simulink model "TD"  (R2018a)
settings: Solver=VariableStepAuto  StartTime=0.0  StopTime=20.0  RelTol=1e-3
libraries: simulink x5
settings Model: Creator=Administrator  LastModifiedBy=Administrator
settings SolverCC: ZeroCrossAlgorithm=Adaptive
settings DebuggingCC: MaxConsecutiveZCsMsg=none  IgnoredZcDiagnostic=none

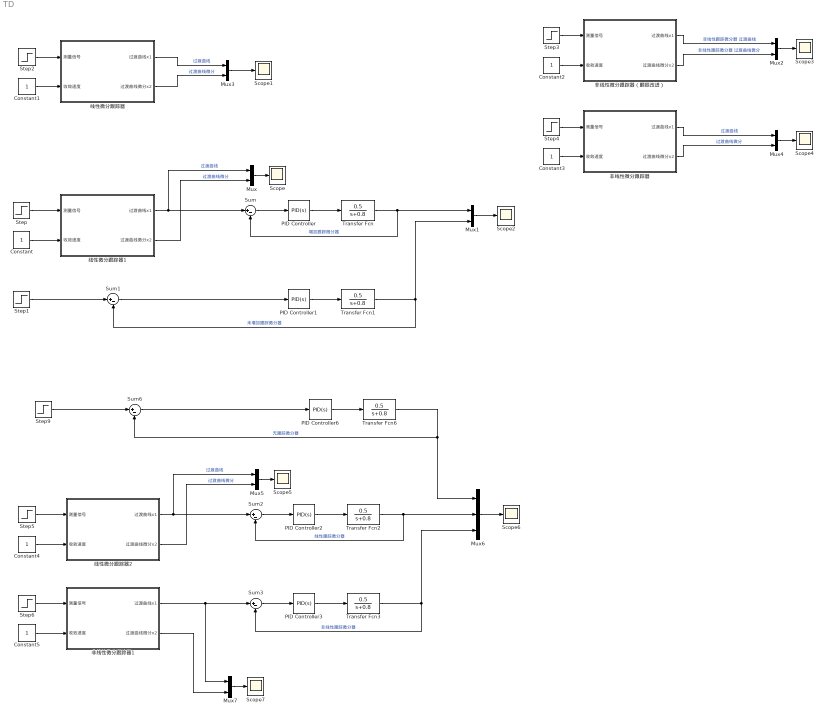
== system TD ==
  Constant{,1..5} (6 alike) : Constant
  Mux{,1..5,7} (7 alike) : Mux  Inputs=2
  Mux6 : Mux  Inputs=3
  PID Controller{,1..3,6} (5 alike) : simulink/Continuous/PID Controller  Controller=PID  TimeDomain=Continuous-time  SampleTime=-1  IntegratorMethod=Forward Euler  FilterMethod=Forward Euler  Form=Parallel  UseFilter=on  ControllerParametersSource=internal  P=10  I=10  D=1  N=100  InitialConditionSource=internal  InitialConditionForIntegrator=0  InitialConditionForFilter=0  ExternalReset=none  LimitOutput=off  UpperSaturationLimit=inf  LowerSaturationLimit=-inf  LinearizeAsGain=on  AntiWindupMode=none  Kb=1  TrackingMode=off  Kt=1  PParamMin=[]  PParamMax=[]  IParamMin=[]  IParamMax=[]  DParamMin=[]  DParamMax=[]  NParamMin=[]  NParamMax=[]  KbParamMin=[]  KbParamMax=[]  KtParamMin=[]  KtParamMax=[]  POutMin=[]  POutMax=[]  IOutMin=[]  IOutMax=[]  DOutMin=[]  DOutMax=[]  NOutMin=[]  NOutMax=[]  KbOutMin=[]  KbOutMax=[]  KtOutMin=[]  KtOutMax=[]  IntegratorOutMin=[]  IntegratorOutMax=[]  FilterOutMin=[]  FilterOutMax=[]  SumOutMin=[]  SumOutMax=[]  SumI1OutMin=[]  SumI1OutMax=[]  SumI2OutMin=[]  SumI2OutMax=[]  SumI3OutMin=[]  SumI3OutMax=[]  SumDOutMin=[]  SumDOutMax=[]  SaturationOutMin=[]  SaturationOutMax=[]  IntegratorContinuousStateAttributes=''  IntegratorStateMustResolveToSignalObject=off  IntegratorRTWStateStorageClass=Auto  FilterContinuousStateAttributes=''  FilterStateMustResolveToSignalObject=off  FilterRTWStateStorageClass=Auto  DifferentiatorICPrevScaledInput=0  DifferentiatorOutMin=[]  DifferentiatorOutMax=[]  FilterDiffOutCoefMin=[]  FilterDiffOutCoefMax=[]  SumDenOutMin=[]  SumDenOutMax=[]  SumNumOutMin=[]  SumNumOutMax=[]  ReciprocalOutMin=[]  ReciprocalOutMax=[]  DivideOutMin=[]  DivideOutMax=[]  TunerSelectOption=Transfer Function Based (PID Tuner App)
  Scope{,1..7} (8 alike) : Scope
  Step{,1..6,9} (8 alike) : Step  SampleTime=0
  Sum{,1..3,6} (5 alike) : Sum  Inputs=|+-
  Transfer Fcn{,1..3,6} (5 alike) : TransferFcn  Numerator=[0.5]  Denominator=[1 0.8]
  线性微分跟踪器 : Subsystem
  线性微分跟踪器1 : Subsystem
  线性微分跟踪器2 : Subsystem
  非线性微分跟踪器 : Subsystem
  非线性微分跟踪器1 : Subsystem
  非线性微分跟踪器（颤振改进） : Subsystem
  wires:
  Step/1 -> 线性微分跟踪器1/1(测量信号)
  Constant/1 -> 线性微分跟踪器1/2(收敛速度)
  线性微分跟踪器1/1(过渡曲线x1) -> Sum/1, Mux/1  "过渡曲线"
  线性微分跟踪器1/2(过渡曲线微分x2) -> Mux/2  "过渡曲线微分"
  Sum/1 -> PID Controller/1
  Mux/1 -> Scope/1
  PID Controller/1 -> Transfer Fcn/1
  PID Controller1/1 -> Transfer Fcn1/1
  Sum1/1 -> PID Controller1/1
  Transfer Fcn/1 -> Sum/2, Mux1/1  "增加跟踪微分器"
  Step2/1 -> 线性微分跟踪器/1(测量信号)
  Constant1/1 -> 线性微分跟踪器/2(收敛速度)
  线性微分跟踪器/1(过渡曲线x1) -> Mux3/1  "过渡曲线"
  线性微分跟踪器/2(过渡曲线微分x2) -> Mux3/2  "过渡曲线微分"
  Mux3/1 -> Scope1/1
  Transfer Fcn1/1 -> Sum1/2, Mux1/2  "未增加跟踪微分器"
  Step1/1 -> Sum1/1
  Mux1/1 -> Scope2/1
  Constant2/1 -> 非线性微分跟踪器（颤振改进）/2(收敛速度)
  Step3/1 -> 非线性微分跟踪器（颤振改进）/1(测量信号)
  Mux2/1 -> Scope3/1
  非线性微分跟踪器（颤振改进）/2(过渡曲线微分x2) -> Mux2/2  "非线性跟踪微分器 过渡曲线微分"
  非线性微分跟踪器（颤振改进）/1(过渡曲线x1) -> Mux2/1  "非线性跟踪微分器 过渡曲线"
  非线性微分跟踪器/1(过渡曲线x1) -> Mux4/1  "过渡曲线"
  非线性微分跟踪器/2(过渡曲线微分x2) -> Mux4/2  "过渡曲线微分"
  Constant3/1 -> 非线性微分跟踪器/2(收敛速度)
  Mux4/1 -> Scope4/1
  Step4/1 -> 非线性微分跟踪器/1(测量信号)
  Constant4/1 -> 线性微分跟踪器2/2(收敛速度)
  Step5/1 -> 线性微分跟踪器2/1(测量信号)
  线性微分跟踪器2/1(过渡曲线x1) -> Sum2/1, Mux5/1  "过渡曲线"
  线性微分跟踪器2/2(过渡曲线微分x2) -> Mux5/2  "过渡曲线微分"
  Mux6/1 -> Scope6/1
  PID Controller2/1 -> Transfer Fcn2/1
  Transfer Fcn3/1 -> Sum3/2, Mux6/3  "非线性跟踪微分器"
  Sum2/1 -> PID Controller2/1
  Sum3/1 -> PID Controller3/1
  PID Controller3/1 -> Transfer Fcn3/1
  Transfer Fcn2/1 -> Sum2/2, Mux6/2  "线性跟踪微分器"
  非线性微分跟踪器1/1(过渡曲线x1) -> Mux7/1, Sum3/1
  Mux5/1 -> Scope5/1
  Step6/1 -> 非线性微分跟踪器1/1(测量信号)
  Constant5/1 -> 非线性微分跟踪器1/2(收敛速度)
  非线性微分跟踪器1/2(过渡曲线微分x2) -> Mux7/2
  Mux7/1 -> Scope7/1
  Sum6/1 -> PID Controller6/1
  PID Controller6/1 -> Transfer Fcn6/1
  Transfer Fcn6/1 -> Mux6/1, Sum6/2  "无跟踪微分器"
  Step9/1 -> Sum6/1

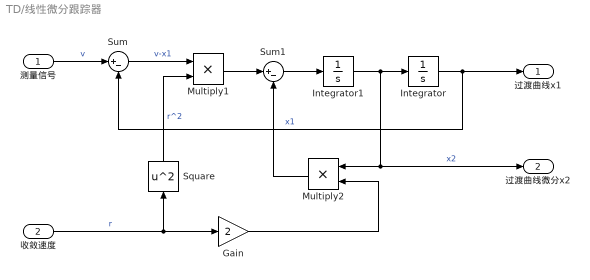
== system TD/线性微分跟踪器 ==
  测量信号 : Inport
  收敛速度 : Inport  Port=2
  Gain : Gain  Gain=2
  Integrator : Integrator
  Integrator1 : Integrator
  Multiply1 : Product
  Multiply2 : Product
  Square : Math  Operator=square  SaturateOnIntegerOverflow=on
  Sum : Sum  Inputs=|+-
  Sum1 : Sum  Inputs=|+-
  过渡曲线x1 : Outport
  过渡曲线微分x2 : Outport  Port=2
  wires:
  Integrator/1 -> 过渡曲线x1/1, Sum/2  "x1"
  Multiply2/1 -> Sum1/2
  Integrator1/1 -> Integrator/1, Multiply2/1, 过渡曲线微分x2/1  "x2"
  测量信号/1 -> Sum/1  "v"
  Multiply1/1 -> Sum1/1
  Sum1/1 -> Integrator1/1
  Gain/1 -> Multiply2/2
  Sum/1 -> Multiply1/1  "v-x1"
  收敛速度/1 -> Square/1, Gain/1  "r"
  Square/1 -> Multiply1/2  "r^2"

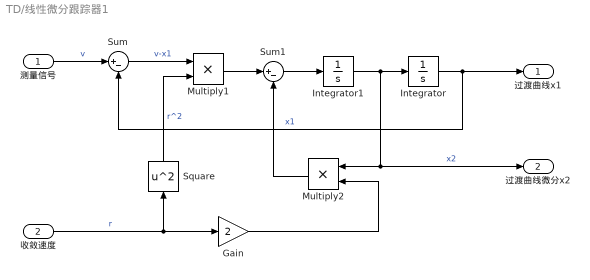
== system TD/线性微分跟踪器1 ==
  测量信号 : Inport
  收敛速度 : Inport  Port=2
  Gain : Gain  Gain=2
  Integrator : Integrator
  Integrator1 : Integrator
  Multiply1 : Product
  Multiply2 : Product
  Square : Math  Operator=square  SaturateOnIntegerOverflow=on
  Sum : Sum  Inputs=|+-
  Sum1 : Sum  Inputs=|+-
  过渡曲线x1 : Outport
  过渡曲线微分x2 : Outport  Port=2
  wires:
  Integrator/1 -> 过渡曲线x1/1, Sum/2  "x1"
  Multiply2/1 -> Sum1/2
  Integrator1/1 -> Integrator/1, Multiply2/1, 过渡曲线微分x2/1  "x2"
  测量信号/1 -> Sum/1  "v"
  Multiply1/1 -> Sum1/1
  Sum1/1 -> Integrator1/1
  Gain/1 -> Multiply2/2
  Sum/1 -> Multiply1/1  "v-x1"
  收敛速度/1 -> Square/1, Gain/1  "r"
  Square/1 -> Multiply1/2  "r^2"

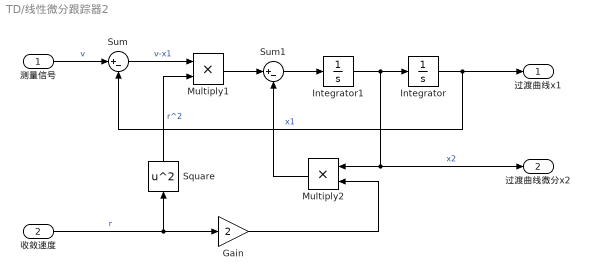
== system TD/线性微分跟踪器2 ==
  测量信号 : Inport
  收敛速度 : Inport  Port=2
  Gain : Gain  Gain=2
  Integrator : Integrator
  Integrator1 : Integrator
  Multiply1 : Product
  Multiply2 : Product
  Square : Math  Operator=square  SaturateOnIntegerOverflow=on
  Sum : Sum  Inputs=|+-
  Sum1 : Sum  Inputs=|+-
  过渡曲线x1 : Outport
  过渡曲线微分x2 : Outport  Port=2
  wires:
  Integrator/1 -> 过渡曲线x1/1, Sum/2  "x1"
  Multiply2/1 -> Sum1/2
  Integrator1/1 -> Integrator/1, Multiply2/1, 过渡曲线微分x2/1  "x2"
  测量信号/1 -> Sum/1  "v"
  Multiply1/1 -> Sum1/1
  Sum1/1 -> Integrator1/1
  Gain/1 -> Multiply2/2
  Sum/1 -> Multiply1/1  "v-x1"
  收敛速度/1 -> Square/1, Gain/1  "r"
  Square/1 -> Multiply1/2  "r^2"

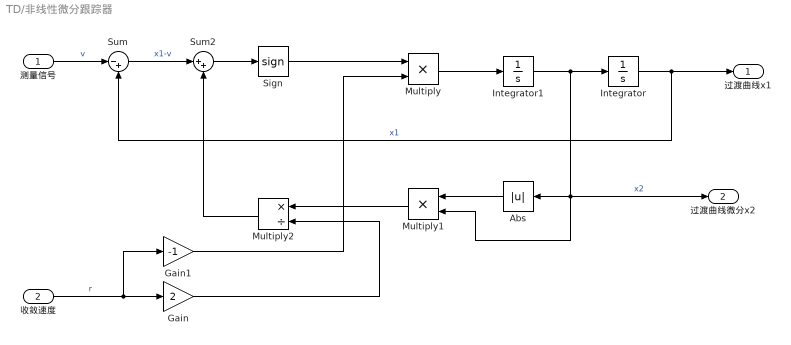
== system TD/非线性微分跟踪器 ==
  测量信号 : Inport
  收敛速度 : Inport  Port=2
  Abs : Abs
  Gain : Gain  Gain=2
  Gain1 : Gain  Gain=-1
  Integrator : Integrator
  Integrator1 : Integrator
  Multiply : Product
  Multiply1 : Product
  Multiply2 : Product  Inputs=*/
  Sign : Signum
  Sum : Sum  Inputs=|-+
  Sum2 : Sum  Inputs=|++
  过渡曲线x1 : Outport
  过渡曲线微分x2 : Outport  Port=2
  wires:
  Integrator/1 -> 过渡曲线x1/1, Sum/2  "x1"
  Multiply2/1 -> Sum2/2
  Integrator1/1 -> Integrator/1, Abs/1, Multiply1/2, 过渡曲线微分x2/1  "x2"
  测量信号/1 -> Sum/1  "v"
  Multiply/1 -> Integrator1/1
  Gain/1 -> Multiply2/2
  Sum/1 -> Sum2/1  "x1-v"
  收敛速度/1 -> Gain/1, Gain1/1  "r"
  Sum2/1 -> Sign/1
  Sign/1 -> Multiply/1
  Gain1/1 -> Multiply/2
  Abs/1 -> Multiply1/1
  Multiply1/1 -> Multiply2/1

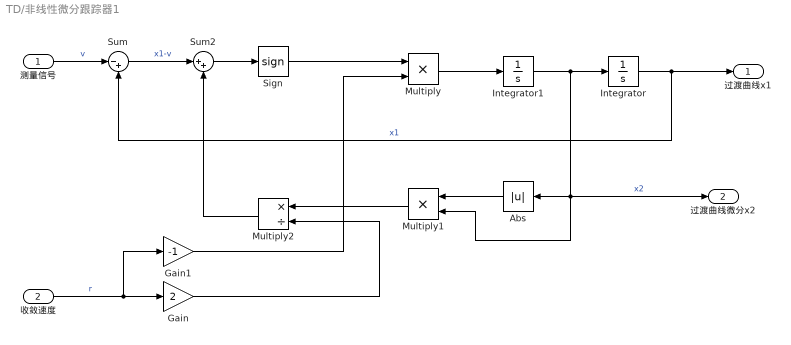
== system TD/非线性微分跟踪器1 ==
  测量信号 : Inport
  收敛速度 : Inport  Port=2
  Abs : Abs
  Gain : Gain  Gain=2
  Gain1 : Gain  Gain=-1
  Integrator : Integrator
  Integrator1 : Integrator
  Multiply : Product
  Multiply1 : Product
  Multiply2 : Product  Inputs=*/
  Sign : Signum
  Sum : Sum  Inputs=|-+
  Sum2 : Sum  Inputs=|++
  过渡曲线x1 : Outport
  过渡曲线微分x2 : Outport  Port=2
  wires:
  Integrator/1 -> 过渡曲线x1/1, Sum/2  "x1"
  Multiply2/1 -> Sum2/2
  Integrator1/1 -> Integrator/1, Abs/1, Multiply1/2, 过渡曲线微分x2/1  "x2"
  测量信号/1 -> Sum/1  "v"
  Multiply/1 -> Integrator1/1
  Gain/1 -> Multiply2/2
  Sum/1 -> Sum2/1  "x1-v"
  收敛速度/1 -> Gain/1, Gain1/1  "r"
  Sum2/1 -> Sign/1
  Sign/1 -> Multiply/1
  Gain1/1 -> Multiply/2
  Abs/1 -> Multiply1/1
  Multiply1/1 -> Multiply2/1

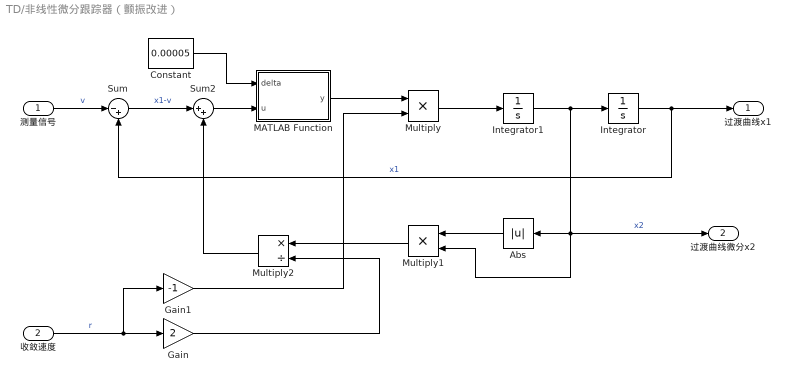
== system TD/非线性微分跟踪器（颤振改进） ==
  测量信号 : Inport
  收敛速度 : Inport  Port=2
  Abs : Abs
  Constant : Constant  Value=0.00005
  Gain : Gain  Gain=2
  Gain1 : Gain  Gain=-1
  Integrator : Integrator
  Integrator1 : Integrator
  MATLAB Function : MATLAB Function  TreatAsAtomicUnit=on
  Multiply : Product
  Multiply1 : Product
  Multiply2 : Product  Inputs=*/
  Sum : Sum  Inputs=|-+
  Sum2 : Sum  Inputs=|++
  过渡曲线x1 : Outport
  过渡曲线微分x2 : Outport  Port=2
  wires:
  Integrator/1 -> 过渡曲线x1/1, Sum/2  "x1"
  Multiply2/1 -> Sum2/2
  Integrator1/1 -> Integrator/1, Abs/1, Multiply1/2, 过渡曲线微分x2/1  "x2"
  测量信号/1 -> Sum/1  "v"
  Multiply/1 -> Integrator1/1
  Gain/1 -> Multiply2/2
  Sum/1 -> Sum2/1  "x1-v"
  收敛速度/1 -> Gain/1, Gain1/1  "r"
  Sum2/1 -> MATLAB Function/2(u)
  MATLAB Function/1(y) -> Multiply/1
  Gain1/1 -> Multiply/2
  Abs/1 -> Multiply1/1
  Multiply1/1 -> Multiply2/1
  Constant/1 -> MATLAB Function/1(delta)

== matlab function TD/非线性微分跟踪器（颤振改进）/MATLAB Function ==
  data: delta input; u input; y output
function y = Saturation(delta, u)

if abs(u) > delta
    y = sign(u);
else
    y = u / delta;
end

end
